simulink model "Lab2_1_sim_2014b"  (R2014b)
settings: Solver=ode45  StartTime=0.0  StopTime=10.0  RelTol=1e-3
settings Model: CovSFcnEnable=on  Creator=Yash Bansod  LastModifiedBy=Yash Bansod
settings DataIOCC: SaveFormat=StructureWithTime
settings DebuggingCC: SolverPrmCheckMsg=none  FrameProcessingCompatibilityMsg=error
settings HardwareCC: ProdBitPerPointer=64  ProdLargestAtomicFloat=Float  ProdIntDivRoundTo=Zero  ProdEndianess=LittleEndian  ProdHWDeviceType=Specified
settings GRTTargetCC: GeneratePreprocessorConditionals=Use local settings

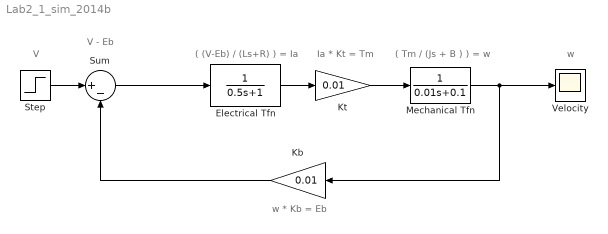
== system Lab2_1_sim_2014b ==
  note: w
  note: V - Eb
  note: V
  note: w * Kb = Eb
  note: ( Tm / (Js + B ) ) = w
  note: Ia * Kt = Tm
  note: ( (V-Eb) / (Ls+R) ) = Ia
  Electrical Tfn : TransferFcn  Denominator=[0.5 1]
  Kb : Gain  Gain=0.01
  Kt : Gain  Gain=0.01
  "Mechanical Tfn " : TransferFcn  Denominator=[0.01 0.1]
  Step : Step  After=220  SampleTime=0
  Sum : Sum  Inputs=|+-
  Velocity : Scope
      settings: TimeRange=auto  MaxDataPoints=5000  SaveToWorkspace=off  SaveName=ScopeData  YMin=-2.74725  YMax=24.72527  SampleTime=-1
  wires:
  Sum/1 -> Electrical Tfn/1
  Step/1 -> Sum/1
  Electrical Tfn/1 -> Kt/1
  Kt/1 -> "Mechanical Tfn "/1
  "Mechanical Tfn "/1 -> Velocity/1, Kb/1
  Kb/1 -> Sum/2
